simulink model "PMSM_sin_hf_vs_test"  (R2022a)
settings: Solver=FixedStepAuto  StartTime=0.0  StopTime=5  FixedStep=1e-4  RelTol=1e-4
model workspace (MAT data in the model file):
  f = Simulink.Signal
  f.DataType = 'single'
  f.Dimensions = 1
  f.DimensionsMode = 'auto'
  f.Complexity = 'real'
  f.SampleTime = -1
  f.SamplingMode = 'auto'
  f.InitialValue = '0.1827'
values from neighbouring files (symbols this model uses):
  curr_d_ki = 35.0    [PMSM_sin_hf_vs.sldd]
  curr_d_kp = 0.17    [PMSM_sin_hf_vs.sldd]
  flux = 0.016884    [PMSM_sin_hf_vs.sldd]
  G1 = -4000.0    [PMSM_sin_hf_vs.sldd]
  G2 = 14000.0    [PMSM_sin_hf_vs.sldd]
  L = 0.00535    [PMSM_sin_hf_vs.sldd]
  Pn = 4.0    [PMSM_sin_hf_vs.sldd]
  Rs = 6.97    [PMSM_sin_hf_vs.sldd]
  spd_ki = 0.0144    [PMSM_sin_hf_vs.sldd]
  spd_kp = 0.3389    [PMSM_sin_hf_vs.sldd]
  Tpwm = 16000.0    [PMSM_sin_hf_vs.sldd]
  Ts = 0.0001    [PMSM_sin_hf_vs.sldd]
  Udc = 24.0    [PMSM_sin_hf_vs.sldd]
undefined symbols (not defined in the file or in its folder): curr_q_ki, curr_q_kp, DiscIntNeverNeededParam, K_Speed_Rate
libraries: slpidlib x4, mcbplantlib x1, simulink x1, autolibpmsmexterior x1
settings Model: DataDictionary=PMSM_sin_hf_vs.sldd  PacingRate=0.630000  Creator=张豪  LastModifiedBy=Administrator
settings OptimizationCC: DefaultParameterBehavior=Inlined  UseDivisionForNetSlopeComputation=on  GainParamInheritBuiltInType=on  UseFloatMulNetSlope=on  InlineInvariantSignals=on  PassReuseOutputArgsAs=Individual arguments  ZeroExternalMemoryAtStartup=off  ZeroInternalMemoryAtStartup=off  NoFixptDivByZeroProtection=on  EfficientFloat2IntCast=on  LifeSpan=1  OptimizeBlockOrder=speed  DifferentSizesBufferReuse=on  EfficientTunableParamExpr=on
settings DebuggingCC: ParameterTunabilityLossMsg=error  UnconnectedInputMsg=warning  UnconnectedOutputMsg=warning  UnconnectedLineMsg=warning
settings HardwareCC: ProdBitPerPointer=32  ProdBitPerSizeT=32  ProdBitPerPtrDiffT=32  ProdLargestAtomicInteger=Long  ProdLargestAtomicFloat=Double  ProdWordSize=32  ProdLongLongMode=on  ProdHWDeviceType=ARM Compatible->ARM Cortex-M
settings SFSimCC: MATLABDynamicMemAlloc=off
settings RTWCC: SystemTargetFile=ert.tlc  GenCodeOnly=on  TemplateMakefile=ert_default_tmf  GenerateReport=on  LaunchReport=on  GenerateCodeReplacementReport=on  DLArmComputeVersion=19.05
settings CodeAppCC: ForceParamTrailComments=on  IgnoreCustomStorageClasses=off  OperatorAnnotations=on  SimulinkDataObjDesc=on  SFDataObjDesc=on  CustomSymbolStrGlobalVar=rt$N$M  CustomSymbolStrType=$N$M  CustomSymbolStrFcn=$N$M$F  CustomSymbolStrMacro=$N$M  InsertBlockDesc=on
settings ERTTargetCC: TargetLangStandard=C99 (ISO)  CodeReplacementLibrary=ARM Cortex-M  GenerateSampleERTMain=on  IncludeMdlTerminateFcn=off  CombineSignalStateStructs=on  SupportComplex=off  SupportNonInlinedSFcns=on  InlinedParameterPlacement=NonHierarchical  ERTCustomFileTemplate=example_file_process.tlc  ERTFilePackagingFormat=CompactWithDataFile

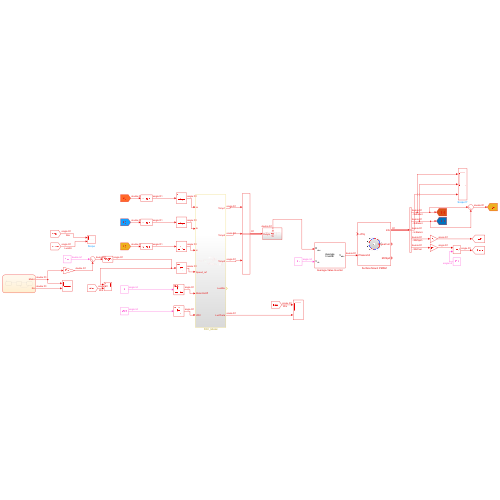
[thumbnail: Simulink's stored preview of the top-level diagram]
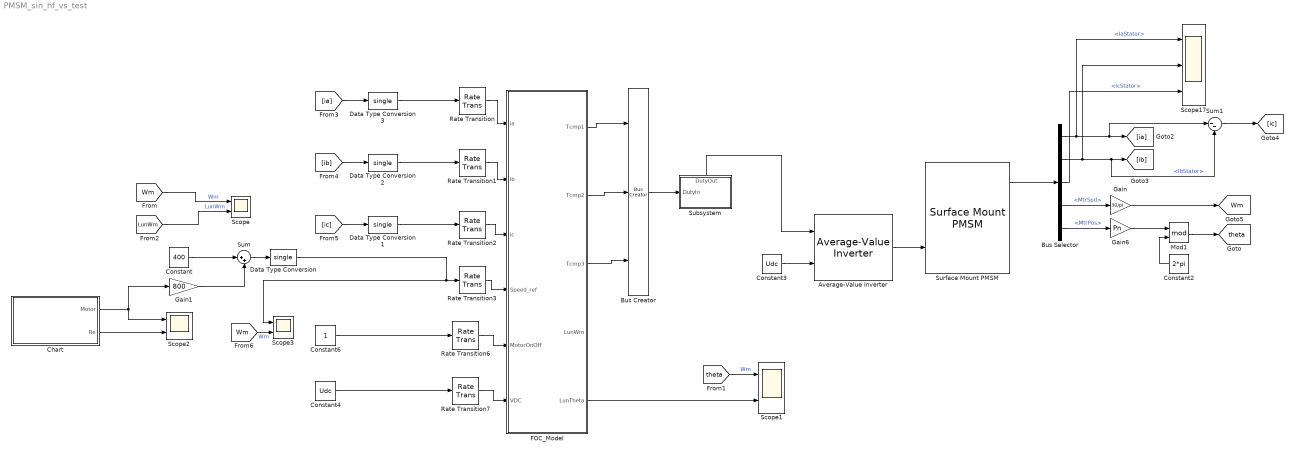
== system PMSM_sin_hf_vs_test ==
  Average-Value Inverter : mcbplantlib/Average-Value Inverter
  Bus Creator : BusCreator  Inputs=3
  Bus Selector : BusSelector  OutputSignals=IaStator,IbStator,IcStator,MtrSpd,MtrPos
  Chart : Stateflow chart  TreatAsAtomicUnit=on
  Constant : Constant  Value=400
  Constant2 : Constant  Value=2*pi  OutDataTypeStr=single
  Constant3 : Constant  Value=Udc
  Constant4 : Constant  Value=Udc  OutDataTypeStr=single
  Constant6 : Constant  OutDataTypeStr=single
  Data Type Conversion{,1..3} (4 alike) : DataTypeConversion  OutDataTypeStr=single  SaturateOnIntegerOverflow=off  RndMeth=Floor
  FOC_Model : Subsystem  SystemSampleTime=5e-5
  Gain : Gain  Gain=30/pi  OutDataTypeStr=single
  Gain1 : Gain  Gain=800
  Gain6 : Gain  Gain=Pn  OutDataTypeStr=single
  Mod1 : Math  Operator=mod  OutputSignalType=real
  Rate Transition{,1..3,6..7} (6 alike) : RateTransition
  Scope{,1..3} (4 alike) : Scope  NumInputPorts=2
  Scope17 : Scope  NumInputPorts=3
  Subsystem : Subsystem
      settings: PortSchema="{\"entries\":[{\"content\":{\"sides\":[{\"content\":{\"connectorIds\":[\"In1\"]},\"type\":\"ConnectorPlacement.EquallySpacedRectSide\",\"uuid\":\"8ccc51de-fa2a-4900-80a3-4cdf9aa76f01\"},{\"content\":{\"connectorIds\":[],\"side\":\"RIGHT\"},\"type\":\"ConnectorPlacement.EquallySpacedRectSide\",\"uuid\":\"32c06e0d-3f1d-4948-af96-e310e54308a0\"},{\"content\":{\"connectorIds\":[\"Out1\"],\"side\":\"TOP\"},\"type\":\"ConnectorPlacement.EquallySpacedRectSide\",\"uuid\":\"a9066067-2c54-42a8-b4d7-fb86ac71b860\"}]},\"type\":\"ConnectorPlacement.EquallySpacedConnector\",\"uuid\":\"e4576975-acad-4e16-822f-2c2e7f23d7a7\"}],\"packageUris\":[\"http://schema.mathworks.com/mf0/Connector/R2020b\"],\"version\":\"1.0\"}"
  Sum : Sum  Inputs=|++
  Sum1 : Sum  Inputs=|--
  Surface Mount PMSM : autolibpmsmexterior/Surface Mount PMSM  port_config=Torque  sim_type=Discrete  Ts=1e-4  P=Pn  Rs=Rs  Ldq_=L  KConstText=Permanent flux linkage constant (lambda_pm):  lambda_pm=flux  Ke=0.0059268  Kt=0.061  mechanical=[75e-6, 8e-5, 0]  idq0=[0 0]  theta_init=4/5  omega_init=0  KConst=flux  lambda_pm_calc=flux  RefBlkName='autolibpmsmexterior/Surface Mount PMSM'  aMode=5  Ldq="[0.0017      0.0017]"
      settings: SourceProductBaseCode=PW,DR,MT,VE
  tag scope: Wm=global, theta=global
  wires:
  Gain/1 -> [Wm]
  [ia] -> Data Type Conversion3/1
  [ib] -> Data Type Conversion2/1
  [ic] -> Data Type Conversion1/1
  Subsystem/1(DutyOut) -> Average-Value Inverter/1
  Average-Value Inverter/1 -> Surface Mount PMSM/2
  Constant3/1 -> Average-Value Inverter/2
  Surface Mount PMSM/1 -> Bus Selector/1
  Bus Selector/1 -> Scope17/1, Sum1/1, [ia]  "<IaStator>"
  Bus Selector/2 -> Scope17/2, [ib], Sum1/2  "<IbStator>"
  Bus Selector/3 -> Scope17/3  "<IcStator>"
  Bus Selector/4 -> Gain/1  "<MtrSpd>"
  Bus Selector/5 -> Gain6/1  "<MtrPos>"
  Bus Creator/1 -> Subsystem/1(DutyIn)
  FOC_Model/1(Tcmp1) -> Bus Creator/1
  FOC_Model/2(Tcmp2) -> Bus Creator/2
  FOC_Model/3(Tcmp3) -> Bus Creator/3
  Data Type Conversion3/1 -> Rate Transition/1
  Data Type Conversion2/1 -> Rate Transition1/1
  Data Type Conversion1/1 -> Rate Transition2/1
  Sum/1 -> Data Type Conversion/1
  Gain6/1 -> Mod1/1
  Constant2/1 -> Mod1/2
  Rate Transition/1 -> FOC_Model/1(ia)
  Rate Transition1/1 -> FOC_Model/2(ib)
  Rate Transition2/1 -> FOC_Model/3(ic)
  Rate Transition3/1 -> FOC_Model/4(Speed_ref)
  Constant4/1 -> Rate Transition7/1
  Rate Transition6/1 -> FOC_Model/5(MotorOnOff)
  Rate Transition7/1 -> FOC_Model/6(VDC)
  Constant6/1 -> Rate Transition6/1
  Mod1/1 -> [theta]
  [Wm] -> Scope/1  "Wm"
  [LunWm] -> Scope/2  "LunWm"
  Chart/1(Motor) -> Gain1/1, Scope2/1
  Chart/2(Re) -> Scope2/2
  FOC_Model/5(LunTheta) -> Scope1/2
  [theta] -> Scope1/1  "Wm"
  Gain1/1 -> Sum/2
  Constant/1 -> Sum/1
  [Wm] -> Scope3/2  "Wm"
  Data Type Conversion/1 -> Scope3/1, Rate Transition3/1
  Sum1/1 -> [ic]

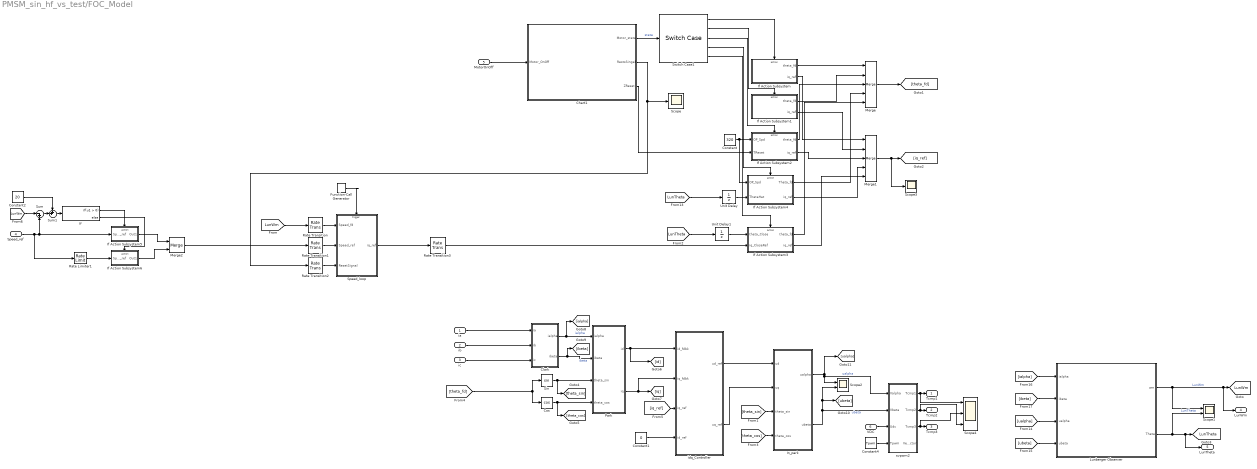
== system PMSM_sin_hf_vs_test/FOC_Model ==
  ia : Inport
  ib : Inport  Port=2
  ic : Inport  Port=3
  Speed_ref : Inport  Port=4
  MotorOnOff : Inport  Port=5
  VDC : Inport  Port=6
  Chart1 : Stateflow chart  TreatAsAtomicUnit=on
  Clark : Subsystem  TreatAsAtomicUnit=on
  Constant : Constant  Value=320  OutDataTypeStr=int32
  Constant1 : Constant  Value=0  OutDataTypeStr=single
  Constant2 : Constant  Value=20
  Constant4 : Constant  Value=Tpwm  OutDataTypeStr=single
  Cos : Trigonometry  Operator=cos
  Function-Call Generator : simulink/Ports & Subsystems/Function-Call Generator  sample_time=1e-3  numberOfIterations=1  DisallowWideOutput=off
  If : If
  If Action Subsystem : Subsystem  TreatAsAtomicUnit=on
  If Action Subsystem1 : Subsystem  TreatAsAtomicUnit=on
  If Action Subsystem2 : Subsystem  TreatAsAtomicUnit=on
  If Action Subsystem3 : Subsystem  TreatAsAtomicUnit=on
  If Action Subsystem4 : Subsystem  TreatAsAtomicUnit=on
  If Action Subsystem5 : Subsystem  TreatAsAtomicUnit=on
  If Action Subsystem6 : Subsystem  TreatAsAtomicUnit=on
  In_park : Subsystem  TreatAsAtomicUnit=on
  Lunberger Observer : Subsystem
  Merge : Merge  Inputs=5
  Merge1 : Merge  Inputs=5
  Merge2 : Merge
  Park : Subsystem  TreatAsAtomicUnit=on
  Rate Limiter1 : RateLimiter  RisingSlewLimit=K_Speed_Rate  FallingSlewLimit=-K_Speed_Rate  SampleTimeMode=inherited
  Rate Transition{,1..3} (4 alike) : RateTransition
  Scope : Scope
  Scope1 : Scope  NumInputPorts=2
  Scope2 : Scope  NumInputPorts=2
  Scope3 : Scope
  Scope4 : Scope  NumInputPorts=3
  Sin : Trigonometry
  Speed_loop : Subsystem
  Sum : Sum  Inputs=|-+
  Sum1 : Sum  Inputs=++|
  Switch Case1 : SwitchCase  CaseConditions={1,2,3,4,5}  ShowDefaultCase=off
  Unit Delay : UnitDelay  SampleTime=-1  HasFrameUpgradeWarning=on
  Unit Delay1 : UnitDelay  SampleTime=-1  HasFrameUpgradeWarning=on
  idq_Controller : Subsystem
  svpwm2 : MATLAB Function  TreatAsAtomicUnit=on
  Tcmp1 : Outport
  Tcmp2 : Outport  Port=2
  Tcmp3 : Outport  Port=3
  LunWm : Outport  Port=4
  LunTheta : Outport  Port=5
  tag scope: LunTheta=global, LunWm=global
  wires:
  MotorOnOff/1 -> Chart1/1(Motor_OnOff)
  Rate Transition/1 -> Speed_loop/1(Speed_fd)
  Rate Transition1/1 -> Speed_loop/2(Speed_ref)
  Rate Transition2/1 -> Speed_loop/3(ResetSignal)
  Chart1/2(RestsSingal) -> Rate Transition2/1, Scope/1
  [LunWm] -> Rate Transition/1
  Function-Call Generator/1 -> Speed_loop/Trigger
  Speed_loop/1(iq_ref) -> Rate Transition3/1
  Constant1/1 -> idq_Controller/4(id_ref)
  svpwm2/2(Tcmp2) -> Tcmp2/1, Scope4/3
  [theta_cos] -> In_park/4(theta_cos)
  If Action Subsystem2/2(iq_ref) -> Merge1/3
  [ualpha] -> Lunberger Observer/3(ualpha)
  svpwm2/1(Tcmp1) -> Tcmp1/1, Scope4/1
  [ibeta] -> Lunberger Observer/2(ibeta)
  In_park/1(ualpha) -> Scope2/1, svpwm2/1(Valpha), [ualpha]  "ualpha"
  [ialpha] -> Lunberger Observer/1(ialpha)
  [LunTheta] -> Unit Delay1/1
  Switch Case1/1 -> If Action Subsystem/Action
  [LunTheta] -> Unit Delay/1
  Lunberger Observer/2(Theta) -> Scope1/2, LunTheta/1, [LunTheta]  "LunTheta"
  If Action Subsystem4/2(iq_ref) -> Merge1/4
  If Action Subsystem3/1(theta_fd) -> Merge/5
  [theta_sin] -> In_park/3(theta_sin)
  Clark/2(ibeta) -> [ibeta], Park/2(ibeta)  "ibeta"
  If Action Subsystem3/2(iq_ref) -> Merge1/5
  Park/2(iq) -> idq_Controller/2(iq_fdbk), [iq]
  In_park/2(ubeta) -> Scope2/2, [ubeta], svpwm2/2(Vbeta)  "ubeta"
  Switch Case1/4 -> If Action Subsystem4/Action
  If Action Subsystem/2(iq_ref) -> Merge1/1
  Park/1(id) -> idq_Controller/1(id_fdbk), [id]
  Merge1/1 -> Scope3/1, [iq_ref]
  Merge/1 -> [theta_fd]
  Rate Transition3/1 -> If Action Subsystem3/2(iq_CloseRef)
  If Action Subsystem1/2(iq_ref) -> Merge1/2
  Cos/1 -> [theta_cos], Park/4(theta_cos)
  If Action Subsystem2/1(theta_fd) -> Merge/3
  If Action Subsystem/1(theta_fd) -> Merge/1
  Switch Case1/2 -> If Action Subsystem1/Action
  Switch Case1/3 -> If Action Subsystem2/Action
  Sin/1 -> Park/3(theta_sin), [theta_sin]
  Unit Delay1/1 -> If Action Subsystem3/1(theta_Close)
  Switch Case1/5 -> If Action Subsystem3/Action
  Constant4/1 -> svpwm2/4(Tpwm)
  Chart1/1(Motor_state) -> Switch Case1/1  "state"
  Chart1/3(ZReset) -> If Action Subsystem2/2(TReset)
  Clark/1(ialpha) -> [ialpha], Park/1(ialpha)  "ialpha"
  If Action Subsystem1/1(theta_fd) -> Merge/2
  If Action Subsystem4/1(Theta_fd) -> Merge/4
  [ubeta] -> Lunberger Observer/4(ubeta)
  Constant/1 -> If Action Subsystem4/1(OP_Spd), If Action Subsystem2/1(OP_Spd)
  Lunberger Observer/1(wm) -> LunWm/1, [LunWm], Scope1/1  "LunWm"
  Unit Delay/1 -> If Action Subsystem4/2(ThetaHat)
  [theta_fd] -> Cos/1, Sin/1
  svpwm2/3(Tcmp3) -> Tcmp3/1, Scope4/2
  VDC/1 -> svpwm2/3(Udc)
  ib/1 -> Clark/2(ib)
  ic/1 -> Clark/3(ic)
  ia/1 -> Clark/1(ia)
  idq_Controller/2(uq_ref) -> In_park/2(uq)
  idq_Controller/1(ud_ref) -> In_park/1(ud)
  [iq_ref] -> idq_Controller/3(iq_ref)
  If/1 -> If Action Subsystem5/Action
  If/2 -> If Action Subsystem6/Action
  If Action Subsystem5/1(Out1) -> Merge2/1
  If Action Subsystem6/1(Out1) -> Merge2/2
  Merge2/1 -> Rate Transition1/1
  Sum/1 -> Sum1/2
  [LunWm] -> Sum/1
  Sum1/1 -> If/1
  Constant2/1 -> Sum1/1
  Speed_ref/1 -> Rate Limiter1/1, If Action Subsystem5/1(Speed_ref), Sum/2
  Rate Limiter1/1 -> If Action Subsystem6/1(Speed_ref)

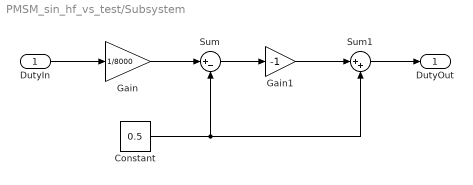
== system PMSM_sin_hf_vs_test/Subsystem ==
  DutyIn : Inport
  Constant : Constant  Value=0.5  SampleTime=-1
  Gain : Gain  Gain=1/8000  ParamDataTypeStr=single
  Gain1 : Gain  Gain=-1
  Sum : Sum  Inputs=|+-
  Sum1 : Sum  Inputs=|++
  DutyOut : Outport
  wires:
  Sum/1 -> Gain1/1
  Constant/1 -> Sum1/2, Sum/2
  DutyIn/1 -> Gain/1
  Gain1/1 -> Sum1/1
  Sum1/1 -> DutyOut/1
  Gain/1 -> Sum/1

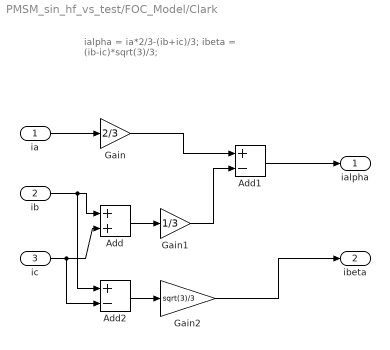
== system PMSM_sin_hf_vs_test/FOC_Model/Clark ==
  note: ialpha = ia*2/3-(ib+ic)/3;
      | ibeta = (ib-ic)*sqrt(3)/3;
  ia : Inport  OutDataTypeStr=single
  ib : Inport  Port=2  OutDataTypeStr=single
  ic : Inport  Port=3  OutDataTypeStr=single
  Add : Sum  AccumDataTypeStr=single  OutDataTypeStr=single
  Add1 : Sum  Inputs=+-  AccumDataTypeStr=single  OutDataTypeStr=single
  Add2 : Sum  Inputs=+-  AccumDataTypeStr=single  OutDataTypeStr=single
  Gain : Gain  Gain=2/3  ParamDataTypeStr=single
  Gain1 : Gain  Gain=1/3  ParamDataTypeStr=single
  Gain2 : Gain  Gain=sqrt(3)/3  ParamDataTypeStr=single
  ialpha : Outport  OutDataTypeStr=single
  ibeta : Outport  Port=2  OutDataTypeStr=single
  wires:
  ia/1 -> Gain/1
  ib/1 -> Add2/1, Add/1
  ic/1 -> Add2/2, Add/2
  Add/1 -> Gain1/1
  Gain/1 -> Add1/1
  Gain1/1 -> Add1/2
  Add1/1 -> ialpha/1
  Add2/1 -> Gain2/1
  Gain2/1 -> ibeta/1

== system PMSM_sin_hf_vs_test/FOC_Model/If Action Subsystem ==
  Action Port : ActionPort  ActionPortLabel=case [ 1 ]:
  Constant : Constant  Value=0  OutDataTypeStr=single
  Constant1 : Constant  Value=0  OutDataTypeStr=single
  theta_fd : Outport
  iq_ref : Outport  Port=2
  wires:
  Constant/1 -> theta_fd/1
  Constant1/1 -> iq_ref/1

== system PMSM_sin_hf_vs_test/FOC_Model/If Action Subsystem1 ==
  Action Port : ActionPort  ActionPortLabel=case [ 2 ]:
  Constant : Constant  Value=0  OutDataTypeStr=single
  Constant1 : Constant  Value=3  OutDataTypeStr=single
  theta_fd : Outport
  iq_ref : Outport  Port=2
  wires:
  Constant1/1 -> iq_ref/1
  Constant/1 -> theta_fd/1

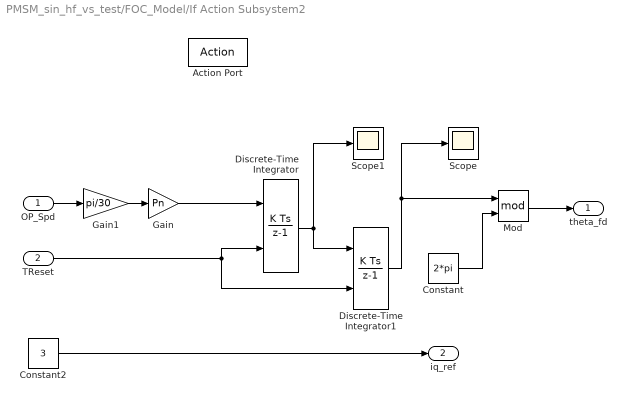
== system PMSM_sin_hf_vs_test/FOC_Model/If Action Subsystem2 ==
  OP_Spd : Inport  OutDataTypeStr=int32  PortDimensions=1
  TReset : Inport  Port=2
  Action Port : ActionPort  ActionPortLabel=case [ 3 ]:
  Constant : Constant  Value=2*pi  OutDataTypeStr=single
  Constant2 : Constant  Value=3  OutDataTypeStr=single
  Discrete-Time Integrator : DiscreteIntegrator  ExternalReset=rising  SampleTime=-1  ICPrevOutput=DiscIntNeverNeededParam  ICPrevScaledInput=DiscIntNeverNeededParam
  Discrete-Time Integrator1 : DiscreteIntegrator  ExternalReset=rising  SampleTime=-1  ICPrevOutput=DiscIntNeverNeededParam  ICPrevScaledInput=DiscIntNeverNeededParam
  Gain : Gain  Gain=Pn
  Gain1 : Gain  Gain=pi/30  OutDataTypeStr=single
  Mod : Math  Operator=mod
  Scope : Scope
  Scope1 : Scope
  theta_fd : Outport
  iq_ref : Outport  Port=2
  wires:
  Gain1/1 -> Gain/1
  Gain/1 -> Discrete-Time Integrator/1
  Constant/1 -> Mod/2
  Discrete-Time Integrator1/1 -> Scope/1, Mod/1
  Mod/1 -> theta_fd/1
  Constant2/1 -> iq_ref/1
  OP_Spd/1 -> Gain1/1
  TReset/1 -> Discrete-Time Integrator/2, Discrete-Time Integrator1/2
  Discrete-Time Integrator/1 -> Scope1/1, Discrete-Time Integrator1/1

== system PMSM_sin_hf_vs_test/FOC_Model/If Action Subsystem3 ==
  theta_Close : Inport
  iq_CloseRef : Inport  Port=2
  Action Port : ActionPort  ActionPortLabel=case [ 5 ]:
  theta_fd : Outport
  iq_ref : Outport  Port=2
  wires:
  iq_CloseRef/1 -> iq_ref/1
  theta_Close/1 -> theta_fd/1

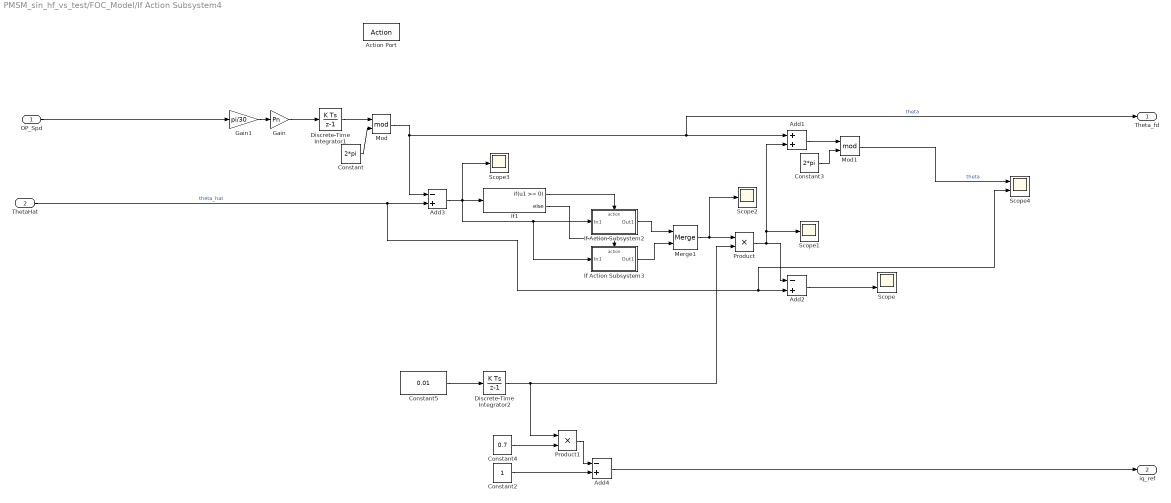
== system PMSM_sin_hf_vs_test/FOC_Model/If Action Subsystem4 ==
  OP_Spd : Inport  OutDataTypeStr=int32  PortDimensions=1
  ThetaHat : Inport  Port=2
  Action Port : ActionPort  ActionPortLabel=case [ 4 ]:
  Add1 : Sum
  Add2 : Sum  Inputs=-+
  Add3 : Sum  Inputs=-+
  Add4 : Sum  Inputs=-+
  Constant : Constant  Value=2*pi  OutDataTypeStr=single
  Constant2 : Constant  OutDataTypeStr=single
  Constant3 : Constant  Value=2*pi  OutDataTypeStr=single
  Constant4 : Constant  Value=0.7  OutDataTypeStr=single
  Constant5 : Constant  Value=0.01  OutDataTypeStr=single
  Discrete-Time Integrator1 : DiscreteIntegrator  SampleTime=-1  ICPrevOutput=DiscIntNeverNeededParam  ICPrevScaledInput=DiscIntNeverNeededParam
  Discrete-Time Integrator2 : DiscreteIntegrator  SampleTime=-1  ICPrevOutput=DiscIntNeverNeededParam  ICPrevScaledInput=DiscIntNeverNeededParam
  Gain : Gain  Gain=Pn
  Gain1 : Gain  Gain=pi/30  OutDataTypeStr=single
  If Action Subsystem2 : Subsystem  TreatAsAtomicUnit=on
  If Action Subsystem3 : Subsystem  TreatAsAtomicUnit=on
  If1 : If  IfExpression=u1 >= 0
  Merge1 : Merge
  Mod : Math  Operator=mod
  Mod1 : Math  Operator=mod
  Product : Product
  Product1 : Product
  Scope : Scope  NumInputPorts=2
  Scope1 : Scope
  Scope2 : Scope
  Scope3 : Scope
  Scope4 : Scope  NumInputPorts=2
  Theta_fd : Outport
  iq_ref : Outport  Port=2
  wires:
  Gain/1 -> Discrete-Time Integrator1/1
  Constant/1 -> Mod/2
  Discrete-Time Integrator1/1 -> Mod/1
  OP_Spd/1 -> Gain1/1
  Gain1/1 -> Gain/1
  ThetaHat/1 -> Scope4/2, Add2/2, Add3/2  "theta_hat"
  Mod/1 -> Theta_fd/1, Add1/1, Add3/1  "theta"
  Add3/1 -> Scope3/1, If Action Subsystem3/1(In1), If Action Subsystem2/1(In1), If1/1
  If1/1 -> If Action Subsystem2/Action
  If1/2 -> If Action Subsystem3/Action
  If Action Subsystem2/1(Out1) -> Merge1/1
  If Action Subsystem3/1(Out1) -> Merge1/2
  Merge1/1 -> Scope2/1, Product/1
  Product/1 -> Add1/2, Scope1/1, Add2/1
  Add2/1 -> Scope/2
  Constant3/1 -> Mod1/2
  Add1/1 -> Mod1/1
  Mod1/1 -> Scope4/1  "theta"
  Constant4/1 -> Product1/2
  Constant2/1 -> Add4/2
  Product1/1 -> Add4/1
  Add4/1 -> iq_ref/1
  Discrete-Time Integrator2/1 -> Product1/1, Product/2
  Constant5/1 -> Discrete-Time Integrator2/1

== system PMSM_sin_hf_vs_test/FOC_Model/If Action Subsystem5 ==
  Speed_ref : Inport
  Action Port : ActionPort  ActionPortLabel=if(u1 > 0)
  Out1 : Outport
  wires:
  Speed_ref/1 -> Out1/1

== system PMSM_sin_hf_vs_test/FOC_Model/If Action Subsystem6 ==
  Speed_ref : Inport
  Action Port : ActionPort  ActionPortLabel=else
  Out1 : Outport
  wires:
  Speed_ref/1 -> Out1/1

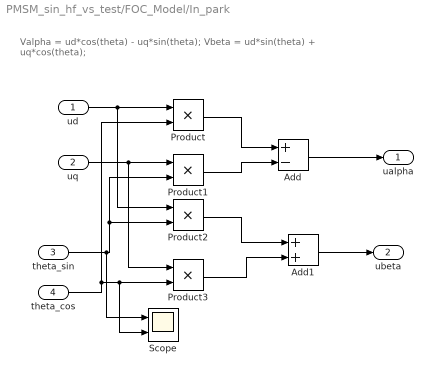
== system PMSM_sin_hf_vs_test/FOC_Model/In_park ==
  note: Valpha = ud*cos(theta) - uq*sin(theta);
      | Vbeta = ud*sin(theta) + uq*cos(theta);
  ud : Inport
  uq : Inport  Port=2
  theta_sin : Inport  Port=3
  theta_cos : Inport  Port=4
  Add : Sum  Inputs=+-
  Add1 : Sum
  Product{,1..3} (4 alike) : Product
  Scope : Scope  NumInputPorts=2
  ualpha : Outport
  ubeta : Outport  Port=2
  wires:
  Add/1 -> ualpha/1
  ud/1 -> Product2/1, Product/1
  theta_cos/1 -> Product/2, Scope/2, Product3/2
  Product/1 -> Add/1
  uq/1 -> Product3/1, Product1/1
  theta_sin/1 -> Scope/1, Product2/2, Product1/2
  Product1/1 -> Add/2
  Product2/1 -> Add1/1
  Product3/1 -> Add1/2
  Add1/1 -> ubeta/1

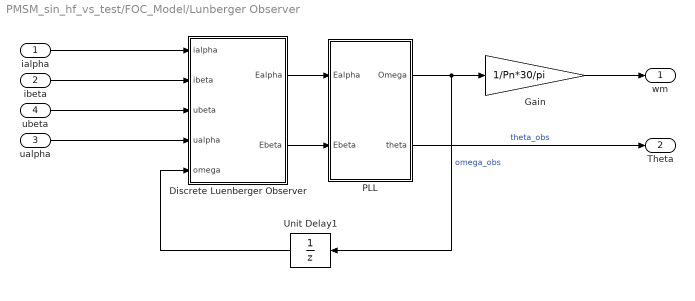
== system PMSM_sin_hf_vs_test/FOC_Model/Lunberger Observer ==
  ialpha : Inport  OutDataTypeStr=single
  ibeta : Inport  Port=2  OutDataTypeStr=single
  ualpha : Inport  Port=3  OutDataTypeStr=single
  ubeta : Inport  Port=4  OutDataTypeStr=single
  Discrete Luenberger Observer : Subsystem
  Gain : Gain  Gain=1/Pn*30/pi  OutDataTypeStr=single
  PLL : Subsystem
  Unit Delay1 : UnitDelay  SampleTime=-1  HasFrameUpgradeWarning=on
  wm : Outport  OutDataTypeStr=single
  Theta : Outport  Port=2  OutDataTypeStr=single
  wires:
  PLL/1(Omega) -> Unit Delay1/1, Gain/1  "omega_obs"
  PLL/2(theta) -> Theta/1  "theta_obs"
  Discrete Luenberger Observer/1(Ealpha) -> PLL/1(Ealpha)
  Discrete Luenberger Observer/2(Ebeta) -> PLL/2(Ebeta)
  ibeta/1 -> Discrete Luenberger Observer/2(ibeta)
  ialpha/1 -> Discrete Luenberger Observer/1(ialpha)
  ualpha/1 -> Discrete Luenberger Observer/4(ualpha)
  ubeta/1 -> Discrete Luenberger Observer/3(ubeta)
  Unit Delay1/1 -> Discrete Luenberger Observer/5(omega)
  Gain/1 -> wm/1

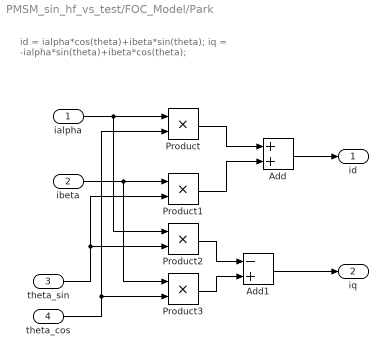
== system PMSM_sin_hf_vs_test/FOC_Model/Park ==
  note: id = ialpha*cos(theta)+ibeta*sin(theta);
      | iq = -ialpha*sin(theta)+ibeta*cos(theta);
  ialpha : Inport  OutDataTypeStr=single
  ibeta : Inport  Port=2  OutDataTypeStr=single
  theta_sin : Inport  Port=3  OutDataTypeStr=single
  theta_cos : Inport  Port=4  OutDataTypeStr=single
  Add : Sum  AccumDataTypeStr=single  OutDataTypeStr=single
  Add1 : Sum  Inputs=-+  AccumDataTypeStr=single  OutDataTypeStr=single
  Product{,1..3} (4 alike) : Product  OutDataTypeStr=single
  id : Outport  OutDataTypeStr=single
  iq : Outport  Port=2  OutDataTypeStr=single
  wires:
  ialpha/1 -> Product2/1, Product/1
  theta_cos/1 -> Product3/2, Product/2
  ibeta/1 -> Product3/1, Product1/1
  theta_sin/1 -> Product2/2, Product1/2
  Product/1 -> Add/1
  Product1/1 -> Add/2
  Add/1 -> id/1
  Product2/1 -> Add1/1
  Product3/1 -> Add1/2
  Add1/1 -> iq/1

== system PMSM_sin_hf_vs_test/FOC_Model/Speed_loop ==
  Speed_fd : Inport  OutDataTypeStr=single  PortDimensions=1
  Speed_ref : Inport  Port=2  OutDataTypeStr=single  PortDimensions=1
  ResetSignal : Inport  Port=3
  Trigger : TriggerPort  TriggerType=function-call  VariantControl=(inherit)  PortDimensions=1
  PID Controller3 : slpidlib/PID Controller  Controller=PI  Form=Parallel  TimeDomain=Discrete-time  UseExternalTs=off  SampleTime=-1  IntegratorMethod=Forward Euler  FilterMethod=Forward Euler  ControllerParametersSource=internal  P=spd_kp  I=spd_ki  UseKiTs=off  D=0  N=100  UseFilter=on  TunerSelectOption=Transfer Function Based (PID Tuner App)  InitialConditionSource=internal  InitialConditionForIntegrator=0  InitialConditionForFilter=0  DifferentiatorICPrevScaledInput=0  ExternalReset=rising  TrackingMode=off  Kt=1  LimitOutput=on  SatLimitsSource=internal  UpperSaturationLimit=3  LowerSaturationLimit=-3  LinearizeAsGain=on  AntiWindupMode=clamping  Kb=0.013  PGainOutDataTypeStr=single  PProdOutDataTypeStr=single  POutMin=[]  POutMax=[]  IGainOutDataTypeStr=single  IProdOutDataTypeStr=single  IOutMin=[]  IOutMax=[]  DOutMin=[]  DOutMax=[]  NOutMin=[]  NOutMax=[]  SumOutDataTypeStr=single  SumOutMin=[]  SumOutMax=[]  SaturationOutDataTypeStr=single  SaturationOutMin=[]  SaturationOutMax=[]  PParamMin=[]  PParamMax=[]  IParamMin=[]  IParamMax=[]  DParamMin=[]  DParamMax=[]  NParamMin=[]  NParamMax=[]  KbParamMin=[]  KbParamMax=[]  KtParamMin=[]  KtParamMax=[]  KbOutMin=[]  KbOutMax=[]  KtOutMin=[]  KtOutMax=[]  IntegratorOutMin=[]  IntegratorOutMax=[]  FilterOutMin=[]  FilterOutMax=[]  SumI1OutMin=[]  SumI1OutMax=[]  SumI2OutMin=[]  SumI2OutMax=[]  SumI3OutMin=[]  SumI3OutMax=[]  SumI4OutMin=[]  SumI4OutMax=[]  SumDOutMin=[]  SumDOutMax=[]  DifferentiatorOutMin=[]  DifferentiatorOutMax=[]  FilterDiffOutCoefMin=[]  FilterDiffOutCoefMax=[]  ReciprocalOutMin=[]  ReciprocalOutMax=[]  SumDenOutMin=[]  SumDenOutMax=[]  SumNumOutMin=[]  SumNumOutMax=[]  DivideOutMin=[]  DivideOutMax=[]  UdiffTsProdOutMin=[]  UdiffTsProdOutMax=[]  NTsProdOutMin=[]  NTsProdOutMax=[]  UintegralTsProdOutMin=[]  UintegralTsProdOutMax=[]  UngainTsProdOutMin=[]  UngainTsProdOutMax=[]  IntegratorContinuousStateAttributes=''  IntegratorStateMustResolveToSignalObject=off  IntegratorRTWStateStorageClass=Auto  FilterContinuousStateAttributes=''  FilterStateMustResolveToSignalObject=off  FilterRTWStateStorageClass=Auto  ParallelPVariant=InternalParameters  IdealPVariant=Disabled  IVariant=InternalParameters  DVariant=Disabled  IntegratorVariant=Discrete  SatVariant=Enabled  AWVariant=DiscClampingParallel  PCopyVariant=Disabled  TRVariant=Disabled  FdbkBlocksVariant=Forward  IdealPFdbkVariant=Disabled  SatFdbkVariant=Disabled  DerivativeFilterVariant=Disabled  NVariant=Disabled  NCopyVariant=Disabled_SignalSpec  FilterICVariant=Disabled  IntegratorICVariant=InternalICs  ExternalResetVariant=ExternalReset  TRSumVariant=Passthrough  SumFdbkVariant=Disabled  SumVariant=Sum_PI  TsampFilterVariant=InternalTs  TsampNgainVariant=Passthrough  TsampIntegralVariant=Passthrough  ExternalSaturationOutDataTypeStr=single  aMode=0
  Sum2 : Sum  Inputs=|+-  AccumDataTypeStr=single  OutDataTypeStr=single
  iq_ref : Outport
  wires:
  Sum2/1 -> PID Controller3/1
  Speed_ref/1 -> Sum2/1
  Speed_fd/1 -> Sum2/2
  PID Controller3/1 -> iq_ref/1
  ResetSignal/1 -> PID Controller3/2

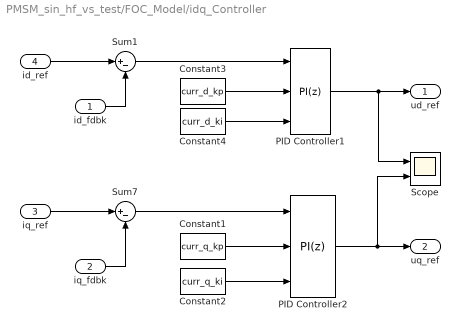
== system PMSM_sin_hf_vs_test/FOC_Model/idq_Controller ==
  id_fdbk : Inport  OutDataTypeStr=single
  iq_fdbk : Inport  Port=2  OutDataTypeStr=single
  iq_ref : Inport  Port=3  OutDataTypeStr=single
  id_ref : Inport  Port=4  OutDataTypeStr=single
  Constant1 : Constant  Value=curr_q_kp  OutDataTypeStr=single
  Constant2 : Constant  Value=curr_q_ki  OutDataTypeStr=single
  Constant3 : Constant  Value=curr_d_kp  OutDataTypeStr=single
  Constant4 : Constant  Value=curr_d_ki  OutDataTypeStr=single
  PID Controller1 : slpidlib/PID Controller  Controller=PI  Form=Parallel  TimeDomain=Discrete-time  UseExternalTs=off  SampleTime=-1  IntegratorMethod=Forward Euler  FilterMethod=Forward Euler  ControllerParametersSource=external  P=curr_d_kp  I=curr_d_ki  UseKiTs=off  D=0  N=100  UseFilter=on  TunerSelectOption=Transfer Function Based (PID Tuner App)  InitialConditionSource=internal  InitialConditionForIntegrator=0  InitialConditionForFilter=0  DifferentiatorICPrevScaledInput=0  ExternalReset=none  TrackingMode=off  Kt=1  LimitOutput=on  SatLimitsSource=internal  UpperSaturationLimit=24*0.9/sqrt(3)  LowerSaturationLimit=-24*0.9/sqrt(3)  LinearizeAsGain=on  AntiWindupMode=clamping  Kb=1  PGainOutDataTypeStr=single  PProdOutDataTypeStr=single  POutMin=[]  POutMax=[]  IGainOutDataTypeStr=int16  IProdOutDataTypeStr=int16  IOutMin=[]  IOutMax=[]  DOutMin=[]  DOutMax=[]  NOutMin=[]  NOutMax=[]  SumOutDataTypeStr=single  SumOutMin=[]  SumOutMax=[]  SaturationOutDataTypeStr=single  SaturationOutMin=[]  SaturationOutMax=[]  PParamMin=[]  PParamMax=[]  IParamMin=[]  IParamMax=[]  DParamMin=[]  DParamMax=[]  NParamMin=[]  NParamMax=[]  KbParamMin=[]  KbParamMax=[]  KtParamMin=[]  KtParamMax=[]  KbOutMin=[]  KbOutMax=[]  KtOutMin=[]  KtOutMax=[]  IntegratorOutMin=[]  IntegratorOutMax=[]  FilterOutMin=[]  FilterOutMax=[]  SumI1OutMin=[]  SumI1OutMax=[]  SumI2OutMin=[]  SumI2OutMax=[]  SumI3OutMin=[]  SumI3OutMax=[]  SumI4OutMin=[]  SumI4OutMax=[]  SumDOutMin=[]  SumDOutMax=[]  DifferentiatorOutMin=[]  DifferentiatorOutMax=[]  FilterDiffOutCoefMin=[]  FilterDiffOutCoefMax=[]  ReciprocalOutMin=[]  ReciprocalOutMax=[]  SumDenOutMin=[]  SumDenOutMax=[]  SumNumOutMin=[]  SumNumOutMax=[]  DivideOutMin=[]  DivideOutMax=[]  UdiffTsProdOutMin=[]  UdiffTsProdOutMax=[]  NTsProdOutMin=[]  NTsProdOutMax=[]  UintegralTsProdOutMin=[]  UintegralTsProdOutMax=[]  UngainTsProdOutMin=[]  UngainTsProdOutMax=[]  IntegratorContinuousStateAttributes=''  IntegratorStateMustResolveToSignalObject=off  IntegratorRTWStateStorageClass=Auto  FilterContinuousStateAttributes=''  FilterStateMustResolveToSignalObject=off  FilterRTWStateStorageClass=Auto  ParallelPVariant=ExternalParameters  IdealPVariant=Disabled  IVariant=ExternalParameters  DVariant=Disabled  IntegratorVariant=Discrete  SatVariant=Enabled  AWVariant=DiscClampingParallel  PCopyVariant=Disabled  TRVariant=Disabled  FdbkBlocksVariant=Forward  IdealPFdbkVariant=Disabled  SatFdbkVariant=Disabled  DerivativeFilterVariant=Disabled  NVariant=Disabled  NCopyVariant=Disabled_SignalSpec  FilterICVariant=Disabled  IntegratorICVariant=InternalICs  ExternalResetVariant=Disabled  TRSumVariant=Passthrough  SumFdbkVariant=Disabled  SumVariant=Sum_PI  TsampFilterVariant=InternalTs  TsampNgainVariant=Passthrough  TsampIntegralVariant=Passthrough  ExternalSaturationOutDataTypeStr=Inherit: Same as second input  aMode=0
  PID Controller2 : slpidlib/PID Controller  Controller=PI  Form=Parallel  TimeDomain=Discrete-time  UseExternalTs=off  SampleTime=-1  IntegratorMethod=Forward Euler  FilterMethod=Forward Euler  ControllerParametersSource=external  P=curr_q_kp  I=curr_q_ki  UseKiTs=off  D=0  N=100  UseFilter=on  TunerSelectOption=Transfer Function Based (PID Tuner App)  InitialConditionSource=internal  InitialConditionForIntegrator=0  InitialConditionForFilter=0  DifferentiatorICPrevScaledInput=0  ExternalReset=none  TrackingMode=off  Kt=1  LimitOutput=on  SatLimitsSource=internal  UpperSaturationLimit=24*0.9/sqrt(3)  LowerSaturationLimit=-24*0.9/sqrt(3)  LinearizeAsGain=on  AntiWindupMode=clamping  Kb=1  PGainOutDataTypeStr=single  PProdOutDataTypeStr=single  POutMin=[]  POutMax=[]  IGainOutDataTypeStr=single  IProdOutDataTypeStr=single  IOutMin=[]  IOutMax=[]  DOutMin=[]  DOutMax=[]  NOutMin=[]  NOutMax=[]  SumOutDataTypeStr=single  SumOutMin=[]  SumOutMax=[]  SaturationOutDataTypeStr=single  SaturationOutMin=[]  SaturationOutMax=[]  PParamMin=[]  PParamMax=[]  IParamMin=[]  IParamMax=[]  DParamMin=[]  DParamMax=[]  NParamMin=[]  NParamMax=[]  KbParamMin=[]  KbParamMax=[]  KtParamMin=[]  KtParamMax=[]  KbOutMin=[]  KbOutMax=[]  KtOutMin=[]  KtOutMax=[]  IntegratorOutMin=[]  IntegratorOutMax=[]  FilterOutMin=[]  FilterOutMax=[]  SumI1OutMin=[]  SumI1OutMax=[]  SumI2OutMin=[]  SumI2OutMax=[]  SumI3OutMin=[]  SumI3OutMax=[]  SumI4OutMin=[]  SumI4OutMax=[]  SumDOutMin=[]  SumDOutMax=[]  DifferentiatorOutMin=[]  DifferentiatorOutMax=[]  FilterDiffOutCoefMin=[]  FilterDiffOutCoefMax=[]  ReciprocalOutMin=[]  ReciprocalOutMax=[]  SumDenOutMin=[]  SumDenOutMax=[]  SumNumOutMin=[]  SumNumOutMax=[]  DivideOutMin=[]  DivideOutMax=[]  UdiffTsProdOutMin=[]  UdiffTsProdOutMax=[]  NTsProdOutMin=[]  NTsProdOutMax=[]  UintegralTsProdOutMin=[]  UintegralTsProdOutMax=[]  UngainTsProdOutMin=[]  UngainTsProdOutMax=[]  IntegratorContinuousStateAttributes=''  IntegratorStateMustResolveToSignalObject=off  IntegratorRTWStateStorageClass=Auto  FilterContinuousStateAttributes=''  FilterStateMustResolveToSignalObject=off  FilterRTWStateStorageClass=Auto  ParallelPVariant=ExternalParameters  IdealPVariant=Disabled  IVariant=ExternalParameters  DVariant=Disabled  IntegratorVariant=Discrete  SatVariant=Enabled  AWVariant=DiscClampingParallel  PCopyVariant=Disabled  TRVariant=Disabled  FdbkBlocksVariant=Forward  IdealPFdbkVariant=Disabled  SatFdbkVariant=Disabled  DerivativeFilterVariant=Disabled  NVariant=Disabled  NCopyVariant=Disabled_SignalSpec  FilterICVariant=Disabled  IntegratorICVariant=InternalICs  ExternalResetVariant=Disabled  TRSumVariant=Passthrough  SumFdbkVariant=Disabled  SumVariant=Sum_PI  TsampFilterVariant=InternalTs  TsampNgainVariant=Passthrough  TsampIntegralVariant=Passthrough  ExternalSaturationOutDataTypeStr=Inherit: Same as second input  aMode=0
  Scope : Scope  NumInputPorts=2
  Sum1 : Sum  Inputs=|+-  AccumDataTypeStr=single  OutDataTypeStr=single
  Sum7 : Sum  Inputs=|+-  AccumDataTypeStr=single  OutDataTypeStr=single
  ud_ref : Outport  OutDataTypeStr=single
  uq_ref : Outport  Port=2  OutDataTypeStr=single
  wires:
  id_fdbk/1 -> Sum1/2
  id_ref/1 -> Sum1/1
  iq_fdbk/1 -> Sum7/2
  Sum1/1 -> PID Controller1/1
  Sum7/1 -> PID Controller2/1
  PID Controller1/1 -> Scope/1, ud_ref/1
  PID Controller2/1 -> Scope/2, uq_ref/1
  iq_ref/1 -> Sum7/1
  Constant3/1 -> PID Controller1/2
  Constant4/1 -> PID Controller1/3
  Constant1/1 -> PID Controller2/2
  Constant2/1 -> PID Controller2/3

== system PMSM_sin_hf_vs_test/FOC_Model/If Action Subsystem4/If Action Subsystem2 ==
  In1 : Inport
  Action Port : ActionPort  ActionPortLabel=if(u1 >= 0)
  Out1 : Outport
  wires:
  In1/1 -> Out1/1

== system PMSM_sin_hf_vs_test/FOC_Model/If Action Subsystem4/If Action Subsystem3 ==
  In1 : Inport
  Action Port : ActionPort  ActionPortLabel=else
  Add : Sum
  Constant : Constant  Value=2*pi  OutDataTypeStr=single
  Out1 : Outport
  wires:
  In1/1 -> Add/1
  Constant/1 -> Add/2
  Add/1 -> Out1/1

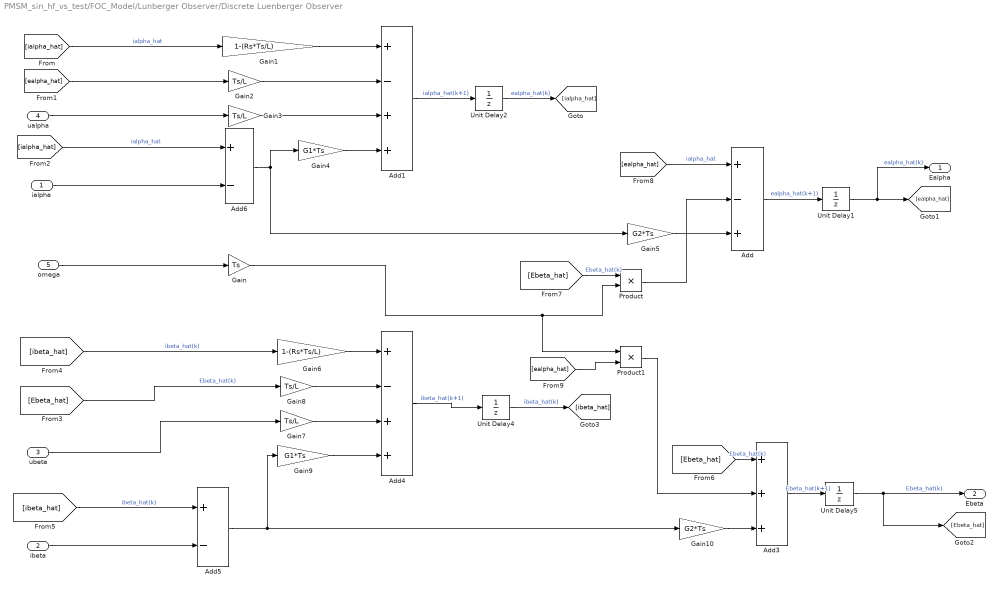
== system PMSM_sin_hf_vs_test/FOC_Model/Lunberger Observer/Discrete Luenberger Observer ==
  ialpha : Inport
  ibeta : Inport  Port=2
  ubeta : Inport  Port=3
  ualpha : Inport  Port=4
  omega : Inport  Port=5
  Add : Sum  Inputs=+-+
  Add1 : Sum  Inputs=+-++
  Add3 : Sum  Inputs=+++
  Add4 : Sum  Inputs=+-++
  Add5 : Sum  Inputs=+-
  Add6 : Sum  Inputs=+-
  Gain : Gain  Gain=Ts
  Gain1 : Gain  Gain=1-(Rs*Ts/L)
  Gain10 : Gain  Gain=G2*Ts
  Gain{2..3,7..8} (4 alike) : Gain  Gain=Ts/L
  Gain4 : Gain  Gain=G1*Ts
  Gain5 : Gain  Gain=G2*Ts
  Gain6 : Gain  Gain=1-(Rs*Ts/L)
  Gain9 : Gain  Gain=G1*Ts
  Product : Product
  Product1 : Product
  Unit Delay{1..2,4..5} (4 alike) : UnitDelay  SampleTime=-1  HasFrameUpgradeWarning=on
  Ealpha : Outport
  Ebeta : Outport  Port=2
  wires:
  Gain8/1 -> Add4/2
  Gain1/1 -> Add1/1
  Add/1 -> Unit Delay1/1  "ealpha_hat(k+1)"
  Add1/1 -> Unit Delay2/1  "ialpha_hat(k+1)"
  Gain2/1 -> Add1/2
  Gain4/1 -> Add1/4
  Gain3/1 -> Add1/3
  ialpha/1 -> Add6/2
  ualpha/1 -> Gain3/1
  omega/1 -> Gain/1
  Gain/1 -> Product/2, Product1/1
  Unit Delay1/1 -> Ealpha/1, [ealpha_hat]  "ealpha_hat(k)"
  Gain5/1 -> Add/3
  Add6/1 -> Gain5/1, Gain4/1
  Unit Delay5/1 -> Ebeta/1, [Ebeta_hat]  "Ebeta_hat(k)"
  Product/1 -> Add/2
  [ialpha_hat] -> Gain1/1  "ialpha_hat"
  Add5/1 -> Gain10/1, Gain9/1
  Gain9/1 -> Add4/4
  ibeta/1 -> Add5/2
  [ibeta_hat] -> Gain6/1  "ibeta_hat(k)"
  Add4/1 -> Unit Delay4/1  "ibeta_hat(k+1)"
  Gain10/1 -> Add3/3
  Add3/1 -> Unit Delay5/1  "Ebeta_hat(k+1)"
  Product1/1 -> Add3/2
  Gain6/1 -> Add4/1
  Gain7/1 -> Add4/3
  ubeta/1 -> Gain7/1
  Unit Delay2/1 -> [ialpha_hat]  "ealpha_hat(k)"
  [ealpha_hat] -> Gain2/1
  [ialpha_hat] -> Add6/1  "ialpha_hat"
  [Ebeta_hat] -> Gain8/1  "Ebeta_hat(k)"
  Unit Delay4/1 -> [ibeta_hat]  "ibeta_hat(k)"
  [ibeta_hat] -> Add5/1  "ibeta_hat(k)"
  [Ebeta_hat] -> Add3/1  "Ebeta_hat(k)"
  [Ebeta_hat] -> Product/1  "Ebeta_hat(k)"
  [ealpha_hat] -> Add/1  "ialpha_hat"
  [ealpha_hat] -> Product1/2

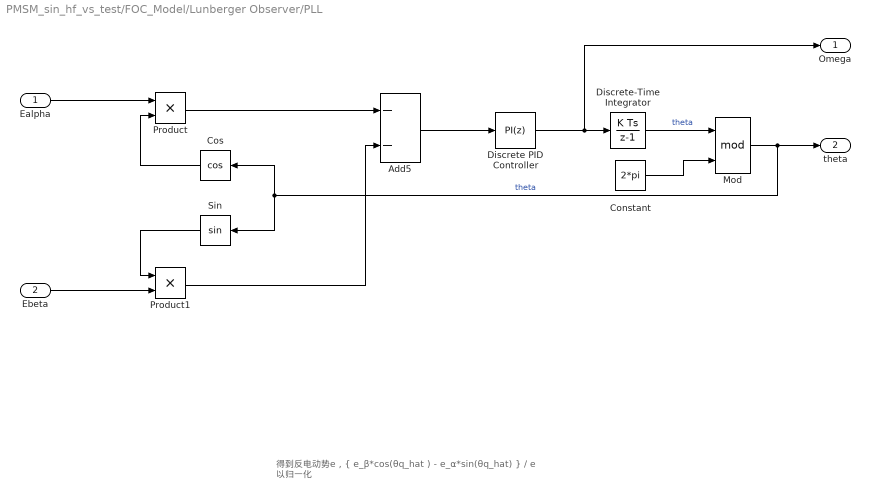
== system PMSM_sin_hf_vs_test/FOC_Model/Lunberger Observer/PLL ==
  note: 得到反电动势e，{ e_β*cos(θq_hat ) - e_α*sin(θq_hat) } / e 以归一化
  Ealpha : Inport  OutDataTypeStr=single
  Ebeta : Inport  Port=2  OutDataTypeStr=single
  Add5 : Sum  Inputs=--  OutDataTypeStr=single
  Constant : Constant  Value=2*pi  OutDataTypeStr=single
  Cos : Trigonometry  Operator=cos
  Discrete PID Controller : slpidlib/PID Controller  Controller=PI  Form=Parallel  TimeDomain=Discrete-time  UseExternalTs=off  SampleTime=-1  IntegratorMethod=Forward Euler  FilterMethod=Forward Euler  ControllerParametersSource=internal  P=2*0.707*150  I=50*50  UseKiTs=off  D=0  N=100  UseFilter=on  TunerSelectOption=Transfer Function Based (PID Tuner App)  InitialConditionSource=internal  InitialConditionForIntegrator=0  InitialConditionForFilter=0  DifferentiatorICPrevScaledInput=0  ExternalReset=none  TrackingMode=off  Kt=1  LimitOutput=on  SatLimitsSource=internal  UpperSaturationLimit=2*pi*1000  LowerSaturationLimit=-2*pi*1000  LinearizeAsGain=on  AntiWindupMode=clamping  Kb=1  POutMin=[]  POutMax=[]  IOutMin=[]  IOutMax=[]  DOutMin=[]  DOutMax=[]  NOutMin=[]  NOutMax=[]  SumOutMin=[]  SumOutMax=[]  SaturationOutMin=[]  SaturationOutMax=[]  PParamMin=[]  PParamMax=[]  IParamMin=[]  IParamMax=[]  DParamMin=[]  DParamMax=[]  NParamMin=[]  NParamMax=[]  KbParamMin=[]  KbParamMax=[]  KtParamMin=[]  KtParamMax=[]  KbOutMin=[]  KbOutMax=[]  KtOutMin=[]  KtOutMax=[]  IntegratorOutMin=[]  IntegratorOutMax=[]  FilterOutMin=[]  FilterOutMax=[]  SumI1OutMin=[]  SumI1OutMax=[]  SumI2OutMin=[]  SumI2OutMax=[]  SumI3OutMin=[]  SumI3OutMax=[]  SumI4OutMin=[]  SumI4OutMax=[]  SumDOutMin=[]  SumDOutMax=[]  DifferentiatorOutMin=[]  DifferentiatorOutMax=[]  FilterDiffOutCoefMin=[]  FilterDiffOutCoefMax=[]  ReciprocalOutMin=[]  ReciprocalOutMax=[]  SumDenOutMin=[]  SumDenOutMax=[]  SumNumOutMin=[]  SumNumOutMax=[]  DivideOutMin=[]  DivideOutMax=[]  UdiffTsProdOutMin=[]  UdiffTsProdOutMax=[]  NTsProdOutMin=[]  NTsProdOutMax=[]  UintegralTsProdOutMin=[]  UintegralTsProdOutMax=[]  UngainTsProdOutMin=[]  UngainTsProdOutMax=[]  IntegratorContinuousStateAttributes=''  IntegratorStateMustResolveToSignalObject=off  IntegratorRTWStateStorageClass=Auto  FilterContinuousStateAttributes=''  FilterStateMustResolveToSignalObject=off  FilterRTWStateStorageClass=Auto  ParallelPVariant=InternalParameters  IdealPVariant=Disabled  IVariant=InternalParameters  DVariant=Disabled  IntegratorVariant=Discrete  SatVariant=Enabled  AWVariant=DiscClampingParallel  PCopyVariant=Disabled  TRVariant=Disabled  FdbkBlocksVariant=Forward  IdealPFdbkVariant=Disabled  SatFdbkVariant=Disabled  DerivativeFilterVariant=Disabled  NVariant=Disabled  NCopyVariant=Disabled_SignalSpec  FilterICVariant=Disabled  IntegratorICVariant=InternalICs  ExternalResetVariant=Disabled  TRSumVariant=Passthrough  SumFdbkVariant=Disabled  SumVariant=Sum_PI  TsampFilterVariant=InternalTs  TsampNgainVariant=Passthrough  TsampIntegralVariant=Passthrough  ExternalSaturationOutDataTypeStr=Inherit: Same as second input  aMode=0
  Discrete-Time Integrator : DiscreteIntegrator  SampleTime=-1  OutDataTypeStr=single  ICPrevOutput=DiscIntNeverNeededParam  ICPrevScaledInput=DiscIntNeverNeededParam
  Mod : Math  Operator=mod
  Product : Product  OutDataTypeStr=single
  Product1 : Product
  Sin : Trigonometry
  Omega : Outport
  theta : Outport  Port=2
  wires:
  Product1/1 -> Add5/2
  Ebeta/1 -> Product1/2
  Sin/1 -> Product1/1
  Ealpha/1 -> Product/1
  Product/1 -> Add5/1
  Mod/1 -> Sin/1, Cos/1, theta/1  "theta"
  Cos/1 -> Product/2
  Discrete PID Controller/1 -> Discrete-Time Integrator/1, Omega/1
  Add5/1 -> Discrete PID Controller/1
  Discrete-Time Integrator/1 -> Mod/1  "theta"
  Constant/1 -> Mod/2

== stateflow chart PMSM_sin_hf_vs_test/Chart ==
  state Motor_HFI1
    en:
    du:
    Motor = 0;
    Re = 0;
  state Motor_InitI
    en:
    du:
    Motor = 0;
    Re = 0;
  state Motor_HFI
    en:
    du:
    Motor = 1;
    Re = 2;
  (default) -> Motor_HFI1
  Motor_HFI1 -> Motor_InitI : [after(5500,tick)]
  Motor_InitI -> Motor_HFI : [after(5000,tick)]
  Motor_HFI -> Motor_InitI : [after(5000,tick)]
  data: Motor output; Re output

== matlab function PMSM_sin_hf_vs_test/FOC_Model/svpwm2 ==
  data: Valpha input; Tcmp1 output; Vbeta input; Udc input; Tpwm input; Tcmp2 output; Tcmp3 output; VecSector output
function [Tcmp1,Tcmp2,Tcmp3,VecSector] = svpwm_(Valpha,Vbeta,Udc,Tpwm) 
Tcmp1=single(0);
Tcmp2=single(0);
Tcmp3=single(0);

T1_tmp = 1.73205078 * Valpha;
VecSector = ((Vbeta + T1_tmp < 0) * 4) + ((T1_tmp > Vbeta) * 2) + (Vbeta > 0); 

T1_tmp = Tpwm/Udc; 

switch VecSector
    case 1
        T1 = (-1.5 * Valpha + 0.866025388 * Vbeta) * T1_tmp;
        Valpha_new = (1.5 * Valpha + 0.866025388 * Vbeta) * T1_tmp;
    case 2
        T1 = (1.5 * Valpha + 0.866025388 * Vbeta) * T1_tmp;
        Valpha_new = -(1.73205078 * Vbeta * T1_tmp);
    case 3
        T1 = -((-1.5 * Valpha + 0.866025388 * Vbeta) * T1_tmp);
        Valpha_new = 1.73205078 * Vbeta * T1_tmp;
    case 4
        T1 = -(1.73205078 * Vbeta * T1_tmp);
        Valpha_new = (-1.5 * Valpha + 0.866025388 * Vbeta) * T1_tmp;
    case 5
        T1 = 1.73205078 * Vbeta * T1_tmp;
        Valpha_new = -((1.5 * Valpha + 0.866025388 * Vbeta) * T1_tmp);
    otherwise
        T1 = -((1.5 * Valpha + 0.866025388 * Vbeta) * T1_tmp);
        Valpha_new = -((-1.5 * Valpha + 0.866025388 * Vbeta) * T1_tmp);
end

% 更新 Valpha
Valpha = Valpha_new;

Vbeta = T1 + Valpha;
if Vbeta > Tpwm
    T1 = T1 / Vbeta;
    Valpha = Valpha / (T1 + Valpha);
end
 
Vbeta = (Tpwm - (T1 + Valpha)) / 4;
T1 = T1 / 2 + Vbeta;
% 循环遍历每个元素

switch VecSector
   case 1
       Tcmp1 = T1; 
       Tcmp2 = Vbeta; 
       Tcmp3 = Valpha / 2 + T1;
   case 2
       Tcmp1 = Vbeta; 
       Tcmp2 = Valpha/ 2 + T1; 
       Tcmp3 = T1;
   case 3
       Tcmp1 = Vbeta; 
       Tcmp2 = T1; 
       Tcmp3 = Valpha / 2 + T1;
   case 4
       Tcmp1 = Valpha / 2 + T1; 
       Tcmp2 = T1; 
       Tcmp3 = Vbeta;
   case 5
       Tcmp1 = Valpha / 2 + T1; 
       Tcmp2 = Vbeta; 
       Tcmp3 = T1;
   case 6
       Tcmp1 = T1; 
       Tcmp2 = Valpha / 2 + T1; 
       Tcmp3 = Vbeta;
end
% [Tcmp1,Tcmp2,Tcmp3]
end

== stateflow chart PMSM_sin_hf_vs_test/FOC_Model/Chart1 ==
  state OpenStage
    en:
    ZReset = 0;
    cnt = 0;
    du:
    if cnt == 1
    ZReset = 1;
    end
    cnt = 1;
    Motor_state = 3;
    RestsSingal = 0;
  state IDLE
    en:
    du:
    Motor_state = 1;
    RestsSingal = 0;
  state AlignStage
    en:
    du:
    Motor_state = 2;
    RestsSingal = 0;
  state ThetaAlign
    en:
    du:
    Motor_state = 4;
    RestsSingal = 0;
  state RunStage
    en:
    du:
    Motor_state = 5;
    RestsSingal = 1;
  (default) -> IDLE
  IDLE -> AlignStage : [Motor_OnOff ==1]
  AlignStage -> OpenStage [order 1] : [after(100,tick)]
  OpenStage -> ThetaAlign [order 2] : [after(10000,tick) ]
  ThetaAlign -> RunStage : [after(10,tick)]
  AlignStage -> IDLE [order 2] : [Motor_OnOff == 0]
  RunStage -> IDLE : [Motor_OnOff ==0]
  OpenStage -> IDLE [order 1] : [Motor_OnOff ==0]
  data: Motor_OnOff input; Motor_state output single; RestsSingal output; ZReset output single; cnt local single
